simulink model "mfistg"  (R2025a)
settings: Solver=VariableStepAuto  StartTime=0.0  StopTime=100  RelTol=1e-3
settings Model: DataDictionary=Constants.sldd  Creator=yaremadzulynsky  LastModifiedBy=levirogalla

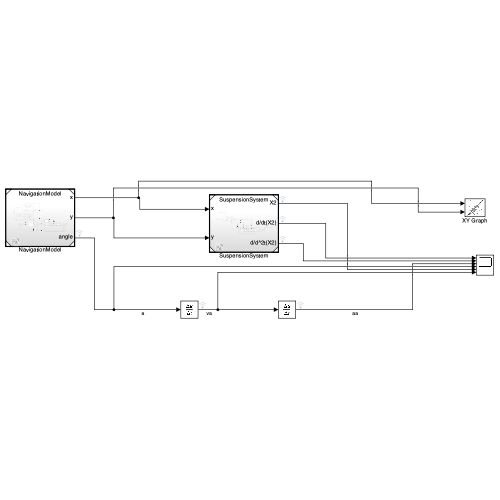
[thumbnail: Simulink's stored preview of the top-level diagram]
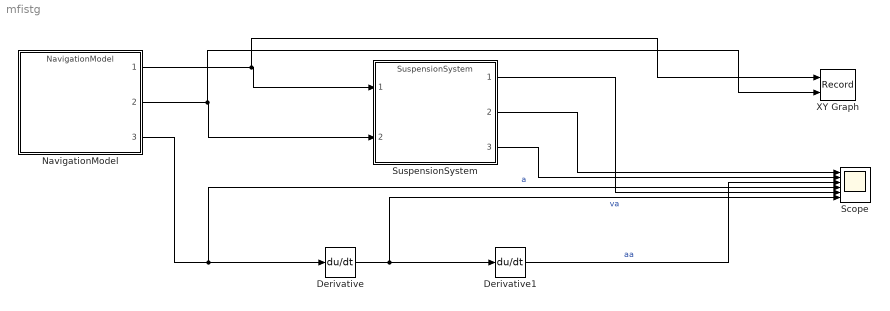
== system mfistg ==
  Derivative : Derivative
  Derivative1 : Derivative
  NavigationModel : ModelReference  ModelNameDialog=NavigationModel.slx  SimulationMode=Normal  ModelReferenceVersion=1.45
  Scope : Scope  NumInputPorts=6
      settings: ActiveDisplayYMinimum=-2.3851103538778955E+8  ActiveDisplayYMaximum=3.0330195973179215E+8
  SuspensionSystem : ModelReference  ModelNameDialog=SuspensionSystem.slx  SimulationMode=Normal  ModelReferenceVersion=1.56
  XY Graph : Record  NumPorts=2.0  FileSettingsInternal="{\"entries\":[{\"content\":{\"excelSettings\":{\"content\":{},\"type\":\"Streamout.ExcelSettings\"},\"parquetSettings\":{\"content\":{},\"type\":\"Streamout.ParquetSettings\"}},\"type\":\"Streamout.FileSettingStorage\",\"uuid\":\"\"}],\"packageUris\":[\"http:\\/\\/schema.mathworks.com\\/mf0\\/streamout_blocks\\/R2020a\"],\"version\":\"1.0\"}"  FrameSettings=[0, 0]  Layout=[1 1]  SignalsInternal="{\"entries\":[{\"content\":{\"signals\":[{\"content\":{\"blockPath\":[],\"dimensions\":[1],\"domain\":\"\",\"lineColor\":\"#a2142f\",\"plots\":[ 1 ],\"port\":1,\"signalID\":1,\"signalName\":\"NavigationModel:1\"},\"type\":\"RecordBlkView.Signal\",\"uuid\":\"\"},{\"content\":{\"blockPath\":[],\"dimensions\":[1],\"domain\":\"\",\"lineColor\":\"#139fff\",\"plots\":[ 1 ],\"port\":2,\"signalID\":2,\"signalName\":\"NavigationModel:2\"},\"type\":\"RecordBlkView.Signal\",\"uuid\":\"\"}]},\"type\":\"RecordBlkView.InputSignals\",\"uuid\":\"\"}],\"packageUris\":[\"http:\\/\\/schema.mathworks.com\\/mf0\\/streamout_blocks\\/R2020a\"],\"version\":\"1.0\"}"  VisualizationBindings="{\"xyplotplugin\":{\"info\":[{\"series\":[{\"bindingParametersList\":[{\"parameter\":\"X-Axis\",\"signalID\":1,\"signalName\":\"NavigationModel:1\"},{\"parameter\":\"Y-Axis\",\"signalID\":2,\"signalName\":\"NavigationModel:2\"}],\"seriesID\":0}],\"subplotID\":1}]}}"  CompatibilityTag=XY
  wires:
  NavigationModel/1 -> XY Graph/1, SuspensionSystem/1
  NavigationModel/2 -> XY Graph/2, SuspensionSystem/2
  SuspensionSystem/1 -> Scope/5
  SuspensionSystem/2 -> Scope/1
  SuspensionSystem/3 -> Scope/2
  NavigationModel/3 -> Scope/4, Derivative/1  "a"
  Derivative/1 -> Scope/6, Derivative1/1  "va"
  Derivative1/1 -> Scope/3  "aa"
